simulink model "SpringDamper_2mass"  (R2017a)
settings: Solver=ode45  StartTime=0.0  StopTime=9.9  RelTol=0.0001
values from neighbouring files (symbols this model uses):
  b1 = .4*Cr    [SeperateVariables_2mass.m]
  b2 = 15002    [SeperateVariables_2mass.m]
  k1 = 400000    [SeperateVariables_2mass.m]
  k2 = 425000    [SeperateVariables_2mass.m]
  m1 = 125    [SeperateVariables_2mass.m]
  m2 = 2.1    [SeperateVariables_2mass.m]
settings Model: Creator=Matthew  LastModifiedBy=Matthew Lemelin

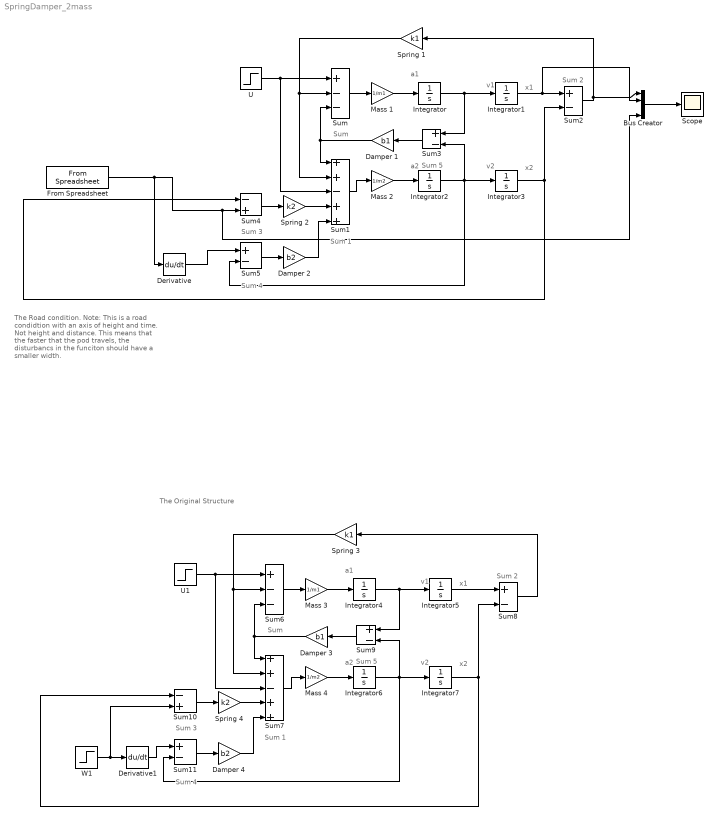
== system SpringDamper_2mass ==
  note: The Road condition. Note: This is a road condidtion with an axis of height and time. Not height and distance. This means that the faster that the pod travels, the disturbancs in the funciton should have a smaller width.
  note: The Original Structure
  note: Sum 3
  note: Sum 4
  note: Sum 5
  note: Sum 2
  note: Sum
  note: Sum 1
  note: a2
  note: v2
  note: x2
  note: x1
  note: v1
  note: a1
  note: Sum 3
  note: Sum 4
  note: Sum 5
  note: Sum 2
  note: Sum
  note: Sum 1
  note: a2
  note: v2
  note: x2
  note: x1
  note: v1
  note: a1
  Bus Creator : BusCreator  Inputs=4
  Damper 1 : Gain  Gain=b1
  Damper 2 : Gain  Gain=b2
  Damper 3 : Gain  Gain=b1
  Damper 4 : Gain  Gain=b2
  Derivative : Derivative
  Derivative1 : Derivative
  From Spreadsheet : FromSpreadsheet  FileName=RoadCondition.xlsx  SheetName=RoadCondition
  Integrator{,1..7} (8 alike) : Integrator
  Mass 1 : Gain  Gain=1/m1
  Mass 2 : Gain  Gain=1/m2
  Mass 3 : Gain  Gain=1/m1
  Mass 4 : Gain  Gain=1/m2
  Scope : Scope
  Spring 1 : Gain  Gain=k1
  Spring 2 : Gain  Gain=k2
  Spring 3 : Gain  Gain=k1
  Spring 4 : Gain  Gain=k2
  Sum : Sum  Inputs=+--
  Sum1 : Sum  Inputs=++-++
  Sum10 : Sum  Inputs=-+
  Sum{2..3,5,8..9,11} (6 alike) : Sum  Inputs=+-
  Sum4 : Sum  Inputs=-+
  Sum6 : Sum  Inputs=+--
  Sum7 : Sum  Inputs=++-++
  U : Step  Time=0  After=0  SampleTime=0
  U1 : Step  Time=0  After=0  SampleTime=0
  W1 : Step  After=0.1  SampleTime=0
  wires:
  Integrator/1 -> Sum3/1, Integrator1/1
  Integrator2/1 -> Sum5/2, Sum3/2, Integrator3/1
  Sum/1 -> Mass 1/1
  Sum1/1 -> Mass 2/1
  Mass 2/1 -> Integrator2/1
  Mass 1/1 -> Integrator/1
  Integrator3/1 -> Sum4/1, Sum2/2
  Integrator1/1 -> Bus Creator/2, Sum2/1
  Sum2/1 -> Bus Creator/1, Spring 1/1
  Spring 1/1 -> Sum1/2, Sum/2
  Sum3/1 -> Damper 1/1
  Damper 1/1 -> Sum/3, Sum1/1
  Sum4/1 -> Spring 2/1
  Spring 2/1 -> Sum1/4
  Damper 2/1 -> Sum1/5
  Sum5/1 -> Damper 2/1
  U/1 -> Sum1/3, Sum/1
  Integrator4/1 -> Sum9/1, Integrator5/1
  Integrator6/1 -> Sum11/2, Sum9/2, Integrator7/1
  Sum6/1 -> Mass 3/1
  Sum7/1 -> Mass 4/1
  Mass 4/1 -> Integrator6/1
  Mass 3/1 -> Integrator4/1
  Integrator7/1 -> Sum10/1, Sum8/2
  Integrator5/1 -> Sum8/1
  Spring 3/1 -> Sum7/2, Sum6/2
  Sum9/1 -> Damper 3/1
  Damper 3/1 -> Sum6/3, Sum7/1
  W1/1 -> Derivative1/1, Sum10/2
  Sum10/1 -> Spring 4/1
  Spring 4/1 -> Sum7/4
  Damper 4/1 -> Sum7/5
  Sum11/1 -> Damper 4/1
  Derivative1/1 -> Sum11/1
  U1/1 -> Sum7/3, Sum6/1
  Sum8/1 -> Spring 3/1
  Bus Creator/1 -> Scope/1
  Derivative/1 -> Sum5/1
  From Spreadsheet/1 -> Derivative/1, Bus Creator/4, Sum4/2
